simulink model "LinearMissileModel"  (R2020b)
settings: Solver=ode4  StartTime=0.0  StopTime=simTime  FixedStep=h  RelTol=1e-3
values from neighbouring files (symbols this model uses):
  N_prime = 4    [LinearizedProNav.m]
  nt = 0    [LinearizedProNav.m]
  Tf = simTime    (= 10)    [LinearizedProNav.m]
  Vc = 4000    [LinearizedProNav.m]
  y = 0    [LinearizedProNav.m]
  yDot = -Vm*HE    (= 60000)    [LinearizedProNav.m]
libraries: simulink x1
settings Model: Creator=dariusmensah  LastModifiedBy=dariusmensah

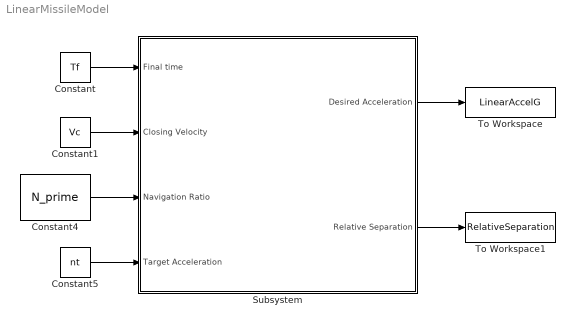
== system LinearMissileModel ==
  Constant : Constant  Value=Tf
  Constant1 : Constant  Value=Vc
  Constant4 : Constant  Value=N_prime
  Constant5 : Constant  Value=nt
  Subsystem : Subsystem
  To Workspace : ToWorkspace  VariableName=LinearAccelG  SaveFormat=Structure With Time  SampleTime=-1
  To Workspace1 : ToWorkspace  VariableName=RelativeSeparation  SaveFormat=Structure With Time  SampleTime=-1
  wires:
  Constant/1 -> Subsystem/1(Final time)
  Constant1/1 -> Subsystem/2(Closing Velocity)
  Constant4/1 -> Subsystem/3(Navigation Ratio)
  Constant5/1 -> Subsystem/4(Target Acceleration)
  Subsystem/1(Desired Acceleration) -> To Workspace/1
  Subsystem/2(Relative Separation) -> To Workspace1/1

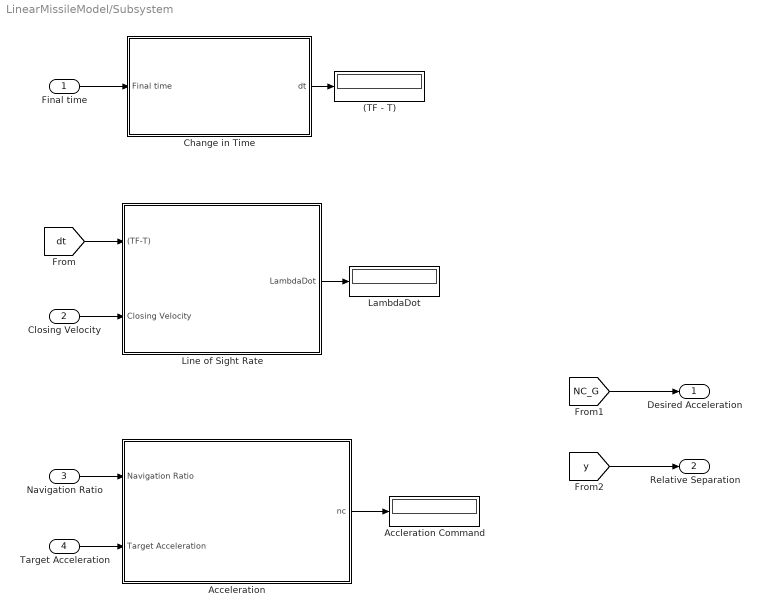
== system LinearMissileModel/Subsystem ==
  Final time : Inport
  Closing Velocity : Inport  Port=2
  Navigation Ratio : Inport  Port=3
  Target Acceleration : Inport  Port=4
  (TF - T) : Display
  Acceleration : Subsystem
  Accleration Command : Display
  Change in Time : Subsystem
  LambdaDot : Display
  Line of Sight Rate : Subsystem
  Desired Acceleration : Outport
  Relative Separation : Outport  Port=2
  wires:
  Final time/1 -> Change in Time/1(Final time)
  Closing Velocity/1 -> Line of Sight Rate/2(Closing Velocity)
  [dt] -> Line of Sight Rate/1((TF-T))
  Change in Time/1(dt) -> (TF - T)/1
  Line of Sight Rate/1(LambdaDot) -> LambdaDot/1
  Navigation Ratio/1 -> Acceleration/1(Navigation Ratio)
  Target Acceleration/1 -> Acceleration/2(Target Acceleration)
  [NC_G] -> Desired Acceleration/1
  Acceleration/1(nc) -> Accleration Command/1
  [y] -> Relative Separation/1

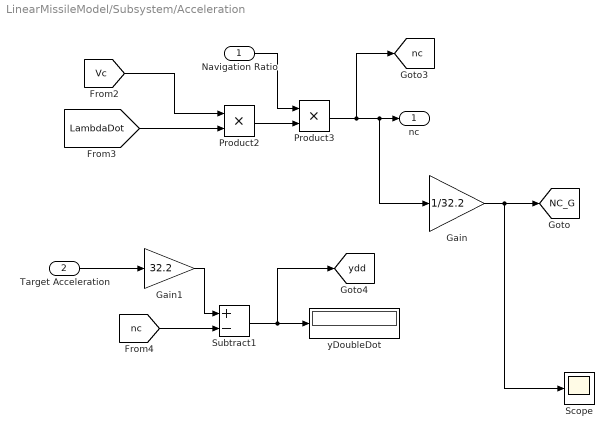
== system LinearMissileModel/Subsystem/Acceleration ==
  Navigation Ratio : Inport
  Target Acceleration : Inport  Port=2
  Gain : Gain  Gain=1/32.2
  Gain1 : Gain  Gain=32.2
  Product2 : Product
  Product3 : Product
  Scope : Scope
  Subtract1 : Sum  Inputs=+-
  yDoubleDot : Display
  nc : Outport
  tag scope: NC_G=global, nc=global, ydd=global
  wires:
  Navigation Ratio/1 -> Product3/1
  [Vc] -> Product2/1
  [LambdaDot] -> Product2/2
  Product2/1 -> Product3/2
  Subtract1/1 -> [ydd], yDoubleDot/1
  [nc] -> Subtract1/2
  Target Acceleration/1 -> Gain1/1
  Product3/1 -> [nc], Gain/1, nc/1
  Gain/1 -> Scope/1, [NC_G]
  Gain1/1 -> Subtract1/1

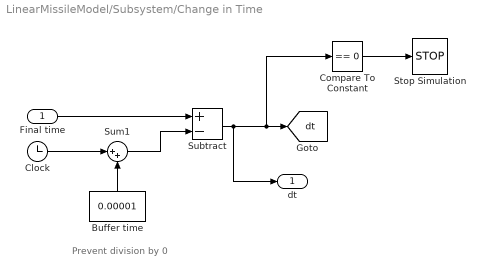
== system LinearMissileModel/Subsystem/Change in Time ==
  note: Prevent division by 0
  Final time : Inport
  Buffer time : Constant  Value=0.00001
  Clock : Clock
  Compare To Constant : simulink/Logic and Bit Operations/Compare To Constant  relop===  const=0  OutDataTypeStr=boolean
  Stop Simulation : Stop
  Subtract : Sum  Inputs=+-
  Sum1 : Sum  Inputs=|++
  dt : Outport
  tag scope: dt=global
  wires:
  Final time/1 -> Subtract/1
  Sum1/1 -> Subtract/2
  Compare To Constant/1 -> Stop Simulation/1
  Buffer time/1 -> Sum1/2
  Subtract/1 -> dt/1, Compare To Constant/1, [dt]
  Clock/1 -> Sum1/1

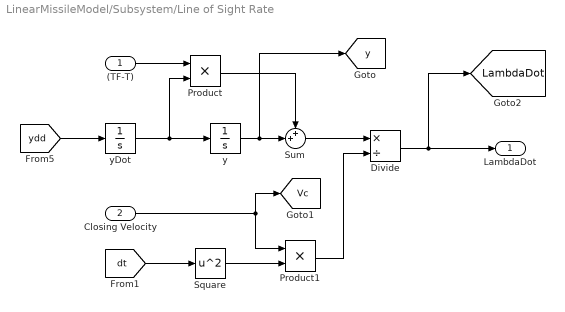
== system LinearMissileModel/Subsystem/Line of Sight Rate ==
  (TF-T) : Inport
  Closing Velocity : Inport  Port=2
  Divide : Product  Inputs=*/
  Product : Product
  Product1 : Product
  Square : Math  Operator=square  SaturateOnIntegerOverflow=on
  Sum : Sum  Inputs=++|
  y : Integrator  InitialCondition=y
  yDot : Integrator  InitialCondition=yDot
  LambdaDot : Outport
  tag scope: LambdaDot=global, Vc=global, y=global
  wires:
  Square/1 -> Product1/2
  Closing Velocity/1 -> [Vc], Product1/1
  Product/1 -> Sum/1
  Sum/1 -> Divide/1
  (TF-T)/1 -> Product/1
  yDot/1 -> Product/2, y/1
  Divide/1 -> LambdaDot/1, [LambdaDot]
  y/1 -> [y], Sum/2
  [dt] -> Square/1
  Product1/1 -> Divide/2
  [ydd] -> yDot/1
